simulink model "practica3"  (R2019b)
settings: Solver=FixedStepAuto  StartTime=0.0  StopTime=10.0  RelTol=1e-3  EnableMultiTasking=on
undefined symbols (not defined in the file or in its folder): Error
libraries: legoev3lib x5
settings Model: ExtModeTrigDuration=2  Creator=alumnopr13  LastModifiedBy=alumnopr13
settings SolverCC: PositivePriorityOrder=on
settings OptimizationCC: EnhancedBackFolding=on  PassReuseOutputArgsAs=Individual arguments  ZeroExternalMemoryAtStartup=off  ZeroInternalMemoryAtStartup=off  MaxStackSize=64  OptimizeBlockOrder=speed  DifferentSizesBufferReuse=on  OptimizationCustomize=off  EfficientTunableParamExpr=on
settings DebuggingCC: ParameterTunabilityLossMsg=error
settings HardwareCC: ProdBitPerPointer=32  ProdBitPerSizeT=32  ProdBitPerPtrDiffT=32  ProdLargestAtomicInteger=Long  ProdWordSize=32  ProdHWDeviceType=ARM Compatible->ARM 9
settings SFSimCC: MATLABDynamicMemAlloc=off
settings RTWCC: SystemTargetFile=ert.tlc  HardwareBoard=LEGO MINDSTORMS EV3  TLCOptions="-aInlineSetEventsForThisBaseRateFcn=TLC_FALSE -aSuppressMultiTaskScheduler=TLC_FALSE  -aRateBasedStepFcn=0"  TemplateMakefile=ert_default_tmf  GenerateReport=on  Toolchain=Sourcery G++ Lite v2009q3  IncludeHyperlinkInReport=on  LaunchReport=on  GenerateTraceInfo=on  GenerateTraceReport=on  GenerateTraceReportSl=on  GenerateTraceReportSf=on  GenerateTraceReportEml=on
settings CodeAppCC: ForceParamTrailComments=on  IgnoreCustomStorageClasses=off  OperatorAnnotations=on  SimulinkDataObjDesc=on  SFDataObjDesc=on  InsertBlockDesc=on
settings ERTTargetCC: SupportContinuousTime=on  SupportVariableSizeSignals=on

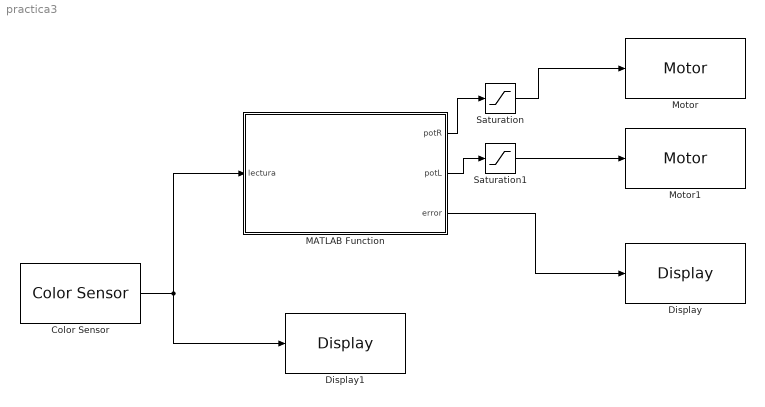
== system practica3 ==
  Color Sensor : legoev3lib/Color Sensor  portNumber=4  mode=Reflected light intensity  sampleTime=0.1
      settings: SourceProductName=Simulink Support Package for LEGO MINDSTORMS EV3 Hardware  SourceProductBaseCode=LEGOEV3
  Display : legoev3lib/Display  slcdStr=Error:  slcdLine=1  slcdFormat=Decimal
      settings: SourceProductName=Simulink Support Package for LEGO MINDSTORMS EV3 Hardware  SourceProductBaseCode=LEGOEV3
  Display1 : legoev3lib/Display  slcdStr=Color  slcdLine=2  slcdFormat=Decimal
      settings: SourceProductName=Simulink Support Package for LEGO MINDSTORMS EV3 Hardware  SourceProductBaseCode=LEGOEV3
  MATLAB Function : MATLAB Function  TreatAsAtomicUnit=on
  Motor : legoev3lib/Motor  sportNumber=A  sstopAction=Brake
  Motor1 : legoev3lib/Motor  sportNumber=D  sstopAction=Brake
  Saturation : Saturate  UpperLimit=20  LowerLimit=-20
  Saturation1 : Saturate  UpperLimit=20  LowerLimit=-20
  wires:
  Color Sensor/1 -> Display1/1, MATLAB Function/1(lectura)
  MATLAB Function/1(potR) -> Saturation/1
  MATLAB Function/2(potL) -> Saturation1/1
  Saturation/1 -> Motor/1
  Saturation1/1 -> Motor1/1
  MATLAB Function/3(error) -> Display/1

== matlab function practica3/MATLAB Function ==
  data: potR output; lectura input; potL output; error output
function[potR, potL, error] = fcn(lectura)
    BLANCO = double(70);
    NEGRO = double(35);
    blanco = double(73);
    negro = double(6);
    persistent int_error;
    persistent ant_error;
    
    if(isempty(int_error))
        int_error = double(0);
    end
    
    if(isempty(ant_error))
        ant_error = double(0);
    end
    
    lectura_recta = double(((lectura-negro)* (BLANCO-NEGRO))/(blanco-negro)+NEGRO);
    error = double(lectura_recta-((BLANCO+NEGRO)/2));
    int_error= int_error + error;
    
    Kp = 0.75;
    Kd = 0.02;
    Ki = 0.08;
    
    G = double((Kp * error) + (Kd * (error - ant_error)) + (Ki * int_error));
    potencia_base = double(10);
	if(error<=-17)
        potR = 0;
        potL = 0;
	elseif(error>=-14)
        potL = 0;
        potR = 0;
    else
        potL =0;
        potR = 0;
    end

    if(G > 30)
       G =  (Kp * error) + (Kd * (error - ant_error));
       int_error = int_error - ant_error;
    end
    
    
    
    
    ant_error = error;
    return
